simulink model "APF_Path_Planning_2023a"  (R2023a)
settings: Solver=ode4  StartTime=0.0  StopTime=tsim  FixedStep=baseRate  RelTol=1e-6  AbsTol=1e-6
values from neighbouring files (symbols this model uses):
  A = [0 0 0 1 0 0 ... (first row only)    [CTL.m]
  a = 25.028    [CTL.m]
  a1 = gain_matrix(1,1)    [CTL.m]
  alpha_m = 0.1    [CTL.m]
  alphap = 1    [CTL.m]
  alphat = 1.1    [CTL.m]
  Am = [0 0 1 0; 0 0 0 1; -wn^2 0 -2*zeta*wn 0; 0 -wn^2 0 -2*zeta*wn]    [CTL.m]
  b = gain_matrix(1,2)    [CTL.m]
  Bm = [0 0; 0 0; -wn^2 0; 0 -wn^2]    [CTL.m]
  c = gain_matrix(2,1)    [CTL.m]
  Cm = [alpha_m 0 0 0; 0 alpha_m 0 0; 0 0 1 0; 0 0 0 1]    [CTL.m]
  d = gain_matrix(2,2)    [CTL.m]
  Dm = zeros(4,2)    [CTL.m]
  epsilon = F_max/2    (= 0.11)    [CTL.m]
  F_max = 0.22    [CTL.m]
  Hz = 0.01    [CTL.m]
  J = IRED    [CTL.m]
  k = lqr(A,B1,Q,R)    [CTL.m]
  k1 = 5    [CTL.m]
  k1t = 2    [CTL.m]
  k2 = 28    [CTL.m]
  k2t = 16    [CTL.m]
  k_1_0 = 3.5    [CTL.m]
  k_1_t_0 = 1    [CTL.m]
  k_2_0 = 28    [CTL.m]
  k_2_t_0 = 1    [CTL.m]
  Kd_t = 9.5    [CTL.m]
  Kd_x = 28    [CTL.m]
  Kd_y = Kd_x    (= 28)    [CTL.m]
  Kp_t = 1    [CTL.m]
  Kp_x = 3.5    [CTL.m]
  Kp_y = Kp_x    (= 3.5)    [CTL.m]
  lambda1 = 0.4    [CTL.m]
  lambda12 = 0.4    [CTL.m]
  lambda12_t = 0.05    [CTL.m]
  lambda1_t = 0.05    [CTL.m]
  lambda2 = 0.4    [CTL.m]
  lambda2_t = 0.05    [CTL.m]
  m = mRED    [CTL.m]
  p = 0.4    [CTL.m]
  p_t = 0.05    [CTL.m]
  Q = [w 0 0 0 0 0 ... (first row only)    [CTL.m]
  R = [r 0 0 ... (first row only)    [CTL.m]
  Red_Rate = 0.025    [CTL.m]
  T_max = 0.0235    [CTL.m]
  Time_Look = 25    [CTL.m]
  xm_0 = [RED_ini(1,1:2),0,0]    [CTL.m]
undefined symbols (not defined in the file or in its folder): a2, a3, adadelta_epsilon, adadelta_gamma, adagrad_epsilon, adagrad_eta, adam_beta_1, adam_beta_2, adam_epsilon, adam_eta, adamax_beta_1, adamax_beta_2, adamax_eta, alpha, Att_Mode, b0, b1, b2, b3, baseRate, beta, Binv, BLACK_end, BLACK_ini, BLUE_end, BLUE_ini, DiscIntNeverNeededParam, drop_states_ARM, drop_states_BLACK, drop_states_BLUE, drop_states_RED, dt, end_time_black, end_time_blue, F_Black_X_nominal, F_Black_Y_nominal, F_Blue_X_nominal, F_Blue_Y_nominal, F_red_X_nominal, F_red_Y_nominal, F_thrusters_BLACK, F_thrusters_BLUE, F_thrusters_RED, Gamma1_el, Gamma1_sh, Gamma1_wr, Gamma2_el, Gamma2_sh, Gamma2_wr, Gamma3_el, Gamma3_sh, Gamma3_wr, Gamma4_el, Gamma4_sh, Gamma4_wr, Gamma5_el, Gamma5_sh, Gamma5_wr, Gamma6_el, Gamma6_sh ... (+98)
libraries: nvidiaSharedBlocks x10, MainLibrary x4, dspsigops x4, simulink x2, etargetslib x1
(part 12 of 13)

== matlab function APF_Path_Planning_2023a/Phase #3: Experiment/Change RED Behavior/Sub-Phase #4/BLACK/UKF1/MATLAB Function ==
  data: Measurments input; States output; Force input; States_k1 input; P_K1 input; P_K output; lamda parameter; J parameter; m parameter; dt parameter; Q parameter; alpha parameter; beta parameter; H parameter; R parameter; thresh parameter
function [States,P_K] = UKF(Measurments,Force,States_k1,P_K1, lamda, J, m, dt, Q, alpha, beta, H, R, thresh)
%% Block diagram got messy so i put it all in one block
if isempty(Force)
    Force = [0;0;0];
end

X_Cal= fcn1(States_k1,P_K1,lamda);

X_Cal_k1 = fcn2(Force,X_Cal,J,m,dt);

[w_m,w_c,X_tilda_k,P_K1] = fcn3(X_Cal_k1,lamda, Q, alpha, beta);

[Z_Bar,Z_Cal] = fcn4(X_Cal_k1, w_m,H);

[P_xz_k,P_z_k] = fcn5(Z_Bar,Z_Cal,w_c,X_tilda_k,X_Cal,R);

K_k = fcn6(P_xz_k,P_z_k);

Z_k = fcn7(Measurments);

Reject = fcn8(Z_k,Z_Bar,P_z_k,thresh);

States = fcn9(Z_k,Reject,X_tilda_k,Z_Bar,K_k);

P_K = fcn10(P_K1,P_z_k,K_k,Reject);
end

function X_Cal = fcn1(x_tilda_k,P_k,lamda)
%% Calculate size of sigma var
sz = 6;
N = 2*sz + 1;
X_Cal = zeros(sz,N);

%% Calculate initial sigma point
X_Cal(:,1) = x_tilda_k;

%% Calculate sigma distance
sigma = (6 + lamda)*P_k;
sigma = Cholesky_Decomposition(sigma);

%% Calculate Sigma Points
% Positive points
for i = 2:1:((N-1)/2) + 1
    fill = zeros(size(x_tilda_k));
    fill(i-1,1) = sigma(i-1,i-1);
    X_Cal(:,i) = x_tilda_k + fill;
end
% Negative Points
j = 1;
for i = N + 1 - ((N-1)/2):1:N
    fill = zeros(size(x_tilda_k));
    fill(j,1) = sigma(j,j);
    X_Cal(:,i) = x_tilda_k - fill;
    j = j + 1;
end
end

function L = Cholesky_Decomposition(mat)
%% Getting size of matrix
[row,col] = size(mat);
%% Make sure matrix can be decomposed
if row ~= col
    disp('Error due to matrix size')
    disp('Make sure square matrix is input into Cholesky Decoposition')
end

if ~isequal(size(mat), size(mat'))
    error('Input matrix must be symmetric');
end

if any(eig(mat) <= 0)
    error('Input matrix must be positive definite');
end

%% Pre allocating Space
L = zeros(row,col);

% Perform Cholesky decomposition
    for i = 1:col
        % Compute the diagonal element
        L(i, i) = sqrt(mat(i, i) - sum(L(i, 1:i-1).^2));
        
        % Compute the elements below the diagonal
        for j = i+1:col
            L(j, i) = (mat(j, i) - sum(L(j, 1:i-1).*L(i, 1:i-1))) / L(i, i);
        end
    end
end

function X_Cal_k1  = fcn2( F, X_Cal_k, J, m, dt)
%% Pre-Define
X_Cal_k1 = zeros(size(X_Cal_k));
%% System Dynamics
A = [eye(3), eye(3)*dt;
    zeros(3), eye(3)];

B = [eye(2)*(dt^2)/(2*m), zeros(2,1);
     0,0, (dt^2)/(2*J);
     eye(2)*(dt)/(m), zeros(2,1);
     0,0, (dt)/(J)];

%% State propigation
f = size(X_Cal_k,2);
for i = 1:1:f
    X_Cal_k1(:,i) = A*X_Cal_k(:,i) + B*F; 
end
end

function [w_m,w_c,X_tilda_k,P_K] = fcn3(X_Cal_k1,lamda, Q, alpha, beta)
%% Sigma weights
sz = size(X_Cal_k1,2);
N = 6;

%% For non modifyed variation
% w_0 = kappa/(N + kappa);
% w_i = 1/(2*(N + kappa));
% w = w_i*ones(1,N);
% w(1,1) = w_0;

%% Additional step - Sigma Points Weights
w_m_0 = lamda/(N + lamda);
w_c_0 = (lamda/(N + lamda)) + beta + (1 - alpha^2);
w_i = 1/(2*(N + lamda));

w = w_i*ones(1,sz-1);
w_m = [w_m_0, w];
w_c = [w_c_0, w];

w_m = diag(w_m);
w_c = diag(w_c);

%% State Prediction
X_tilda_k = X_Cal_k1*w_m;
X_tilda_k = sum(X_tilda_k,2);


%% Covariance Prediction
P_K = (X_Cal_k1 - X_tilda_k)*w_c*(X_Cal_k1 - X_tilda_k)' + Q;

end

function [Z_Bar,Z_Cal] = fcn4(x_Cal_k1, w_m,H)
%% calc Z_Cal
N = size(x_Cal_k1,2);
Z_Cal = zeros(3,N);
for i = 1:1:N
    Z_Cal(:,i) = H*x_Cal_k1(:,i);
end

%% Calc Z_Bar
Z_Bar = Z_Cal*w_m;
Z_Bar = sum(Z_Bar,2);
end

function [P_xz_k,P_z_k] = fcn5(Z_Bar,Z_Cal,w_c,x_tilda_k1,X_Cal,R)
%% calc P_z
P_z_k = (Z_Cal - Z_Bar)*w_c*(Z_Cal - Z_Bar)' + R;

%% calc P_xz
P_xz_k = (X_Cal - x_tilda_k1)*w_c*(Z_Cal - Z_Bar)';
end

function K_k = fcn6(P_xz_k,P_z_k)
K_k = (P_xz_k)*P_z_k';
end

function Z_k = fcn7(z_k)
    %% Assuming that all states are given or no states are given
    if anynan(z_k)
        Z_k = 1000*ones(3,1);
    else
    Z_k = z_k;
    end
end

function  Reject = fcn8(Z_k,Z_Bar,P_z_k,thresh)
%% Calc Mahalanobis Distance
D_square = (transpose(Z_k - Z_Bar))*P_z_k*(Z_k - Z_Bar);
% mahalanobis_d = sqrt(D_square);

%% Determine if data should be rejected
if D_square < thresh
    Reject = 0;
else
    Reject = 1;
end
end

function [x] = fcn9(z,Reject,X_tilda_k,z_bar,K_k)
%% State estimate
    if Reject == 0
        x = X_tilda_k + K_k*(z - z_bar);
    else
        x = X_tilda_k;
    end
end

function P_K = fcn10(P_k1,P_z_k,K_k,Reject)
if Reject == 0
    P_K = P_k1 - (K_k*P_z_k)*K_k';
else
    P_K = P_k1;
end
end

== matlab function APF_Path_Planning_2023a/Phase #3: Experiment/Change BLUE Behavior/Sub-Phase #3 /Hough Control/MATLAB Function2 ==
  data: Oy output; z input; Ox output
function [Oy, Ox]   = C3( z )
%C3 gives the rotation matrix about the z-axis for an angle 'z'
%   z - the angle about the z-axis which you rotate
%   A - the rotation matrix

Ox = [cos(z) sin(z); -sin(z) cos(z)]*[1;0];
Oy = [cos(z) sin(z); -sin(z) cos(z)]*[0;1];
end

== matlab function APF_Path_Planning_2023a/Phase #3: Experiment/Change BLUE Behavior/Sub-Phase #3 /Hough Control/MATLAB Function3 ==
  data: z input; Ox output
function Ox    = C3( z )
%C3 gives the rotation matrix about the z-axis for an angle 'z'
%   z - the angle about the z-axis which you rotate
%   A - the rotation matrix

Ox = [cos(z) sin(z); -sin(z) cos(z)]*[1;0];
end

== matlab function APF_Path_Planning_2023a/Phase #3: Experiment/Change BLUE Behavior/Sub-Phase #3 /Hough Control/MATLAB Function4 ==
  data: Oy input; e_out output; e_in input
function e_out = fcn(Oy, e_in)

a = sign(Oy'*e_in);
e_out = -a*norm(e_in);

== matlab function APF_Path_Planning_2023a/Phase #3: Experiment/Change BLUE Behavior/Sub-Phase #3 /MATLAB Function2 ==
  data: t input; x output; xLength parameter
function x = fcn(t, xLength)

x = -0.85*cos((0.03490659)*t) + xLength/2;

end

== matlab function APF_Path_Planning_2023a/Phase #3: Experiment/Change BLUE Behavior/Sub-Phase #3 /MATLAB Function3 ==
  data: t input; y output; yLength parameter
function y = fcn(t, yLength)

y = -0.85*sin((0.03490659)*t) + yLength/2;

end

== matlab function APF_Path_Planning_2023a/Phase #5: Hold Home/Change BLUE Behavior/Hough Control/MATLAB Function4 ==
  data: Oy input; e_out output; e_in input
function e_out = fcn(Oy, e_in)

a = sign(Oy'*e_in);
e_out = -a*norm(e_in);

== matlab function APF_Path_Planning_2023a/Phase #3: Experiment/Change RED Behavior/Sub-Phase #4/BLACK/Parker's Transform ==
  data: rel_state_black input; state_red input; abs_state_black output
function abs_state_black = fcn(rel_state_black,state_red)
%calcualtes ECI pos/att of black

% messing with rel state black
rel_state_black(1) = rel_state_black(1)/100;
rel_state_black(2) = rel_state_black(2)/100;
rel_state_black(3) = rel_state_black(3)*(pi/180)+pi/2; 

angle = -state_red(3);

C = [cos(angle),sin(angle);
     -sin(angle),cos(angle)];

abs_distance_black = C*[rel_state_black(1);rel_state_black(2)];

abs_pos_black = [state_red(1);state_red(2)] + abs_distance_black;

abs_angle_black = rel_state_black(3) - state_red(3);

abs_state_black =  [abs_pos_black;
                    abs_angle_black];

== matlab function APF_Path_Planning_2023a/Phase #3: Experiment/Change RED Behavior/Sub-Phase #4/BLACK/Kalman Filter1/MATLAB Function ==
  data: z_k input; Z_k output
function Z_k = fcn(z_k)
    %% Assuming that all states are given or no states are given
    if anynan(z_k)
        Z_k = zeros(3,1);
    else
    Z_k = z_k;
    end
end

== matlab function APF_Path_Planning_2023a/Phase #3: Experiment/Change RED Behavior/Sub-Phase #4/BLACK/Kalman Filter1/MATLAB Function1 ==
  data: P_k input; P_k1 output; A parameter; Q_T parameter
function P_k1 = fcn(P_k,A, Q_T)
if isempty(P_k) 
    P_k1 = Peye(6);
else
    P_k1 = A*P_k*(transpose(A)) + Q_T;
end
end

== matlab function APF_Path_Planning_2023a/Phase #3: Experiment/Change RED Behavior/Sub-Phase #4/BLACK/Kalman Filter1/MATLAB Function2 ==
  data: P_k1 input; K_k output; H parameter; R parameter
function K_k = fcn(P_k1,H, R)

K_k = P_k1*(transpose(H))/(H*P_k1*(transpose(H)) + R);
end

== matlab function APF_Path_Planning_2023a/Phase #3: Experiment/Change RED Behavior/Sub-Phase #4/BLACK/Kalman Filter1/MATLAB Function3 ==
  data: P_k1 input; P_K output; K_k input; H parameter
function P_K = fcn(P_k1,K_k,H)
P_K = zeros(6,6);
P_K = P_k1 - (K_k*H*P_k1); 
end

== matlab function APF_Path_Planning_2023a/Phase #3: Experiment/Change RED Behavior/Sub-Phase #4/BLACK/Kalman Filter1/MATLAB Function4 ==
  data: Z_k input; x output; X_tilda_k input; K_k input; H parameter
function x = fcn(Z_k,X_tilda_k,K_k,H)

x = X_tilda_k + K_k*(Z_k - H*X_tilda_k);
end

== matlab function APF_Path_Planning_2023a/Phase #3: Experiment/Change RED Behavior/Sub-Phase #4/BLACK/Kalman Filter1/MATLAB Function5 ==
  data: X_tilda_k1 input; x_tilda_k output; A parameter
function x_tilda_k = fcn(X_tilda_k1,A)

x_tilda_k = A*X_tilda_k1;
end

== matlab function APF_Path_Planning_2023a/Phase #3: Experiment/Change RED Behavior/Sub-Phase #4/CTL/Target Tracker/LQR1/MATLAB Function ==
  data: k input; u output; q1_x input; q2_x input; q1_y input; q2_y input; q1_t input; q2_t input
function u = fcn(k,q1_x,q2_x,q1_y,q2_y,q1_t,q2_t)

x = [q1_x;
    q1_y;
    q1_t;
    q2_x;
    q2_y;
    q2_t];

u = k*x;
% u = [0; 0; 0];

== matlab function APF_Path_Planning_2023a/Phase #3: Experiment/Change RED Behavior/Sub-Phase #4/CTL/If Action Subsystem/CSMC3/MATLAB Function ==
  data: phi input; u output; alphap parameter
function u = fcn(phi, alphap)



u = sign(phi)*(abs(phi)^(alphap/(2 - alphap)));

== matlab function APF_Path_Planning_2023a/Phase #5: Hold Home/Change RED Behavior/Hough Control/MATLAB Function2 ==
  data: Oy output; z input; Ox output
function [Oy, Ox]   = C3( z )
%C3 gives the rotation matrix about the z-axis for an angle 'z'
%   z - the angle about the z-axis which you rotate
%   A - the rotation matrix

Ox = [cos(z) sin(z); -sin(z) cos(z)]*[1;0];
Oy = [cos(z) sin(z); -sin(z) cos(z)]*[0;1];
end

== matlab function APF_Path_Planning_2023a/Phase #3: Experiment/Change RED Behavior/Sub-Phase #4/GDC/Target Finder/Constant Angular Rate/Wrap1/MATLAB Function ==
  data: u input; wrappedAngle output
function wrappedAngle = wrapAngle(u)

wrappedAngle = atan2(sin(u),cos(u));

end

== matlab function APF_Path_Planning_2023a/Phase #3: Experiment/Change RED Behavior/Sub-Phase #4/CTL/If Action Subsystem/CSMC3/MATLAB Function1 ==
  data: q2 input; u output; k1 parameter; alphap parameter
function u = fcn(q2,k1, alphap)

u = sign(k1*q2)*(abs(k1*q2)^alphap);

== matlab function APF_Path_Planning_2023a/Phase #3: Experiment/Change RED Behavior/Sub-Phase #4/CTL/If Action Subsystem/CSMC3/MATLAB Function2 ==
  data: q1 input; phi output; k1 parameter; alphap parameter; q2 input
function phi = fcn(q1,k1, alphap, q2)



phi = k1*q1 + (1/(2 - alphap))*sign(k1*q2)*(abs(k1*q2))^(2 - alphap);

== matlab function APF_Path_Planning_2023a/Phase #3: Experiment/Change RED Behavior/Sub-Phase #4/CTL/If Action Subsystem/CSMC3/MATLAB Function3 ==
  data: phi input; u output; alphap parameter
function u = fcn(phi, alphap)



u = sign(phi)*(abs(phi)^(alphap/(2 - alphap)));

== matlab function APF_Path_Planning_2023a/Phase #3: Experiment/Change RED Behavior/Sub-Phase #4/CTL/If Action Subsystem/CSMC3/MATLAB Function4 ==
  data: q2 input; u output; k1 parameter; alphap parameter
function u = fcn(q2,k1, alphap)

u = sign(k1*q2)*(abs(k1*q2)^alphap);

== matlab function APF_Path_Planning_2023a/Phase #3: Experiment/Change RED Behavior/Sub-Phase #4/CTL/If Action Subsystem/CSMC3/MATLAB Function5 ==
  data: q1 input; phi output; k1 parameter; alphap parameter; q2 input
function phi = fcn(q1,k1, alphap, q2)



phi = k1*q1 + (1/(2 - alphap))*sign(k1*q2)*(abs(k1*q2))^(2 - alphap);

== matlab function APF_Path_Planning_2023a/Phase #3: Experiment/Change RED Behavior/Sub-Phase #4/CTL/If Action Subsystem/CSMC3/MATLAB Function6 ==
  data: phi input; u output; alpha parameter
function u = fcn(phi, alpha)



u = sign(phi)*(abs(phi)^(alpha/(2 - alpha)));

== matlab function APF_Path_Planning_2023a/Phase #3: Experiment/Change RED Behavior/Sub-Phase #4/CTL/If Action Subsystem/CSMC3/MATLAB Function7 ==
  data: q2 input; u output; k1 parameter; alpha parameter
function u = fcn(q2,k1, alpha)

u = sign(k1*q2)*(abs(k1*q2)^alpha);

== matlab function APF_Path_Planning_2023a/Phase #3: Experiment/Change RED Behavior/Sub-Phase #4/CTL/If Action Subsystem/CSMC3/MATLAB Function8 ==
  data: q1 input; phi output; k1 parameter; alpha parameter; q2 input
function phi = fcn(q1,k1, alpha, q2)



phi = k1*q1 + (1/(2 - alpha))*sign(k1*q2)*(abs(k1*q2))^(2 - alpha);

== matlab function APF_Path_Planning_2023a/Phase #5: Hold Home/Change RED Behavior/Hough Control/MATLAB Function3 ==
  data: z input; Ox output
function Ox    = C3( z )
%C3 gives the rotation matrix about the z-axis for an angle 'z'
%   z - the angle about the z-axis which you rotate
%   A - the rotation matrix

Ox = [cos(z) sin(z); -sin(z) cos(z)]*[1;0];
end

== matlab function APF_Path_Planning_2023a/Phase #3: Experiment/Change RED Behavior/Sub-Phase #4/CTL/If Action Subsystem/DAC Controller2/Fx Gain Derivatives ==
  data: e_xdot input; k2_dot output; e_x input; k1_dot output; lambda1 parameter; lambda2 parameter; lambda12 parameter; p parameter
function [k2_dot, k1_dot]= fcn(e_xdot, e_x, lambda1, lambda2, lambda12, p)

k1_dot = -lambda1*p*e_x^2-(lambda1+p*lambda12)*e_x*e_xdot-lambda12*e_xdot^2;
k2_dot = -lambda12*p*e_x^2-(lambda12+p*lambda2)*e_x*e_xdot-lambda2*e_xdot^2;

== matlab function APF_Path_Planning_2023a/Phase #3: Experiment/Change RED Behavior/Sub-Phase #4/CTL/If Action Subsystem/DAC Controller2/Fy Gain Derivatives ==
  data: k2_dot output; e_ydot input; e_y input; k1_dot output; lambda1 parameter; lambda2 parameter; lambda12 parameter; p parameter
function [k2_dot, k1_dot]= fcn(e_ydot, e_y, lambda1, lambda2, lambda12, p)

k1_dot = -lambda1*p*e_y^2-(lambda1+p*lambda12)*e_y*e_ydot-lambda12*e_ydot^2;
k2_dot = -lambda12*p*e_y^2-(lambda12+p*lambda2)*e_y*e_ydot-lambda2*e_ydot^2;

== matlab function APF_Path_Planning_2023a/Phase #3: Experiment/Change RED Behavior/Sub-Phase #4/CTL/If Action Subsystem/DAC Controller2/Torque Gain Derivatives ==
  data: e_t input; e_tdot input; k1_dot output size=1; k2_dot output size=1; lambda1_t parameter; lambda2_t parameter; lambda12_t parameter; p_t parameter
function [k1_dot, k2_dot]= fcn(e_t, e_tdot, lambda1_t, lambda2_t, lambda12_t, p_t)
k1_dot = -lambda1_t*p_t*e_t^2-(lambda1_t+p_t*lambda12_t)*e_t*e_tdot-lambda12_t*e_tdot^2;
k2_dot = -lambda12_t*p_t*e_t^2-(lambda12_t+p_t*lambda2_t)*e_t*e_tdot-lambda2_t*e_tdot^2;

== matlab function APF_Path_Planning_2023a/Phase #3: Experiment/Change RED Behavior/Sub-Phase #4/CTL/If Action Subsystem/Homo/MATLAB Function ==
  data: q1 input; u output; k1 parameter; alphap parameter
function u = fcn(q1,k1, alphap)

u = k1*sign(q1)*(abs(q1)^(alphap/(2 - alphap)));

== matlab function APF_Path_Planning_2023a/Phase #3: Experiment/Change RED Behavior/Sub-Phase #4/CTL/If Action Subsystem/Homo/MATLAB Function1 ==
  data: q2 input; u output; k2 parameter; alphap parameter
function u = fcn(q2,k2, alphap)

u = k2*sign(q2)*(abs(q2)^alphap);

== matlab function APF_Path_Planning_2023a/Phase #3: Experiment/Change RED Behavior/Sub-Phase #4/CTL/If Action Subsystem/DAC Controller1/Fy Gain Derivatives ==
  data: k2_dot output; e_ydot input; e_y input; k1_dot output; lambda1 parameter; lambda2 parameter; lambda12 parameter; p parameter
function [k2_dot, k1_dot]= fcn(e_ydot, e_y, lambda1, lambda2, lambda12, p)

k1_dot = -lambda1*p*e_y^2-(lambda1+p*lambda12)*e_y*e_ydot-lambda12*e_ydot^2;
k2_dot = -lambda12*p*e_y^2-(lambda12+p*lambda2)*e_y*e_ydot-lambda2*e_ydot^2;

== matlab function APF_Path_Planning_2023a/Phase #5: Hold Home/Change RED Behavior/Hough Control/MATLAB Function4 ==
  data: Oy input; e_out output; e_in input
function e_out = fcn(Oy, e_in)

a = sign(Oy'*e_in);
e_out = -a*norm(e_in);

== matlab function APF_Path_Planning_2023a/Phase #3: Experiment/Change RED Behavior/Sub-Phase #4/CTL/If Action Subsystem/DAC Controller1/Torque Gain Derivatives ==
  data: e_t input; e_tdot input; k1_dot output size=1; k2_dot output size=1; lambda1_t parameter; lambda2_t parameter; lambda12_t parameter; p_t parameter
function [k1_dot, k2_dot]= fcn(e_t, e_tdot, lambda1_t, lambda2_t, lambda12_t, p_t)
k1_dot = -lambda1_t*p_t*e_t^2-(lambda1_t+p_t*lambda12_t)*e_t*e_tdot-lambda12_t*e_tdot^2;
k2_dot = -lambda12_t*p_t*e_t^2-(lambda12_t+p_t*lambda2_t)*e_t*e_tdot-lambda2_t*e_tdot^2;

== matlab function APF_Path_Planning_2023a/Phase #3: Experiment/Change RED Behavior/Sub-Phase #4/CTL/If Action Subsystem/Homo/MATLAB Function4 ==
  data: q1 input; u output; k1t parameter; alphat parameter
function u = fcn(q1,k1t, alphat)

u = k1t*sign(q1)*(abs(q1)^(alphat/(2 - alphat)));

== matlab function APF_Path_Planning_2023a/Phase #3: Experiment/Change RED Behavior/Sub-Phase #4/CTL/If Action Subsystem/Homo/MATLAB Function5 ==
  data: q2 input; u output; k2t parameter; alphat parameter
function u = fcn(q2,k2t, alphat)

u = k2t*sign(q2)*(abs(q2)^alphat);

== matlab function APF_Path_Planning_2023a/Phase #3: Experiment/Change RED Behavior/Sub-Phase #4/CTL/If Action Subsystem/LQR/MATLAB Function ==
  data: k input; u output; q1_x input; q2_x input; q1_y input; q2_y input; q1_t input; q2_t input
function u = fcn(k,q1_x,q2_x,q1_y,q2_y,q1_t,q2_t)

x = [q1_x;
    q1_y;
    q1_t;
    q2_x;
    q2_y;
    q2_t];

u = k*x;
% u = [0; 0; 0];

== matlab function APF_Path_Planning_2023a/Phase #3: Experiment/Change RED Behavior/Sub-Phase #4/CTL/If Action Subsystem/Sat/MATLAB Function ==
  data: q2 input; q1 input; saturation output; a1 parameter; b parameter; m parameter
function saturation = fcn(q2,q1,a1, b, m)

u = a1*m*q1 + a1*m*q2/b;

saturation = u;

== matlab function APF_Path_Planning_2023a/Phase #3: Experiment/Change RED Behavior/Sub-Phase #4/CTL/If Action Subsystem/Sat/MATLAB Function1 ==
  data: q2 input; q1 input; saturation output; a1 parameter; b parameter; m parameter
function saturation = fcn(q2,q1,a1, b, m)

u = a1*m*q1 + a1*m*q2/b;

saturation = u;

== matlab function APF_Path_Planning_2023a/Phase #3: Experiment/Change RED Behavior/Sub-Phase #4/CTL/If Action Subsystem/Sat/MATLAB Function2 ==
  data: q2 input; q1 input; saturation output; c parameter; d parameter; J parameter
function saturation = fcn(q2,q1,c, d, J)

u = c*J*q1 + c*J*q2/d;

saturation = u;

== matlab function APF_Path_Planning_2023a/Simulate Plant Dynamics/RED and ARM Dynamics/RED + ARM/RED + ARM Dynamics/Coriolis Function1 ==
  data: a1 parameter; a2 parameter; a3 parameter; b0 parameter; b1 parameter; b2 parameter; mPROX parameter; mDIST parameter; mEE parameter; Phi parameter; CoriolisS output; x input
function CoriolisS = CoriolisFunc3LINK(a1,a2,a3,b0,b1,b2,mPROX,mDIST,mEE,Phi,x)
%CORIOLISFUNC3LINK
%    CORIOLISS = CORIOLISFUNC3LINK(A1,A2,A3,B0,B1,B2,mPROX,mDIST,mEE,PHI,Q0,Q1,Q2,Q3,Q0_DOT,Q1_DOT,Q2_DOT,Q3_DOT)

%    This function was generated by the Symbolic Math Toolbox version 8.0.
%    05-Nov-2017 11:48:44

q0 = x(3);
q1 = x(4);
q2 = x(5);
q3 = x(6);

q0_dot = x(9);
q1_dot = x(10);
q2_dot = x(11);
q3_dot = x(12);

t2 = a1+b1;
t3 = a1.*mPROX;
t4 = mDIST.*t2;
t5 = mEE.*t2;
t6 = t3+t4+t5;
t7 = a2.*mDIST;
t8 = a2+b2;
t9 = mEE.*t8;
t10 = t7+t9;
t11 = pi.*(1.0./2.0);
t12 = q0_dot.*t6;
t13 = q1_dot.*t6;
t14 = q0+q1+t11;
t15 = cos(t14);
t16 = t12+t13;
t17 = q0_dot.*t10;
t18 = q1_dot.*t10;
t19 = q2_dot.*t10;
t20 = q0+q1+q2+t11;
t21 = cos(t20);
t22 = t17+t18+t19;
t23 = a3.*mEE.*q0_dot;
t24 = a3.*mEE.*q1_dot;
t25 = a3.*mEE.*q2_dot;
t26 = a3.*mEE.*q3_dot;
t27 = q0+q1+q2+q3+t11;
t28 = cos(t27);
t29 = t23+t24+t25+t26;
t30 = b0.*mPROX;
t31 = b0.*mDIST;
t32 = b0.*mEE;
t33 = t30+t31+t32;
t34 = (pi/2-Phi)+q0;
t35 = sin(t14);
t36 = sin(t20);
t37 = sin(t27);
t38 = q0_dot+q1_dot+q2_dot+q3_dot;
t39 = q0+q1+q2+q3;
t40 = a1.*b0.*mPROX.*q1_dot;
t41 = a1.*b0.*mDIST.*q1_dot;
t42 = a1.*b0.*mEE.*q1_dot;
t43 = b0.*b1.*mDIST.*q1_dot;
t44 = b0.*b1.*mEE.*q1_dot;
t45 = (pi/2-Phi)-q1;
t46 = cos(t45);
t47 = a2.*b0.*mDIST.*q1_dot;
t48 = a2.*b0.*mDIST.*q2_dot;
t49 = a2.*b0.*mEE.*q1_dot;
t50 = a2.*b0.*mEE.*q2_dot;
t51 = b0.*b2.*mEE.*q1_dot;
t52 = b0.*b2.*mEE.*q2_dot;
t53 = -(pi/2-Phi)+q1+q2;
t54 = cos(t53);
t55 = a3.*b0.*mEE.*q1_dot;
t56 = a3.*b0.*mEE.*q2_dot;
t57 = a3.*b0.*mEE.*q3_dot;
t58 = -(pi/2-Phi)+q1+q2+q3;
t59 = cos(t58);
t60 = a2.*b1.*mDIST.*q2_dot;
t61 = a1.*b2.*mEE.*q2_dot;
t62 = a2.*b1.*mEE.*q2_dot;
t63 = b1.*b2.*mEE.*q2_dot;
t64 = a1.*a2.*mDIST.*q2_dot;
t65 = a1.*a2.*mEE.*q2_dot;
t66 = sin(q2);
t67 = t60+t61+t62+t63+t64+t65;
t68 = a3.*b2.*mEE.*q3_dot;
t69 = a2.*a3.*mEE.*q3_dot;
t70 = sin(q3);
t71 = t68+t69;
t72 = a3.*b1.*mEE.*q2_dot;
t73 = a3.*b1.*mEE.*q3_dot;
t74 = a1.*a3.*mEE.*q2_dot;
t75 = a1.*a3.*mEE.*q3_dot;
t76 = q2+q3;
t77 = sin(t76);
t78 = t72+t73+t74+t75;
t79 = a2.*b0.*mDIST.*q0_dot;
t80 = a2.*b0.*mEE.*q0_dot;
t81 = b0.*b2.*mEE.*q0_dot;
t82 = t47+t48+t49+t50+t51+t52+t79+t80+t81;
t83 = a3.*b0.*mEE.*q0_dot;
t84 = t55+t56+t57+t83;
t85 = a1.*b0.*mPROX.*q0_dot;
t86 = a1.*b0.*mDIST.*q0_dot;
t87 = a1.*b0.*mEE.*q0_dot;
t88 = b0.*b1.*mDIST.*q0_dot;
t89 = b0.*b1.*mEE.*q0_dot;
t90 = a2.*b1.*mDIST.*q0_dot;
t91 = a1.*b2.*mEE.*q0_dot;
t92 = a2.*b1.*mDIST.*q1_dot;
t93 = a2.*b1.*mEE.*q0_dot;
t94 = a1.*b2.*mEE.*q1_dot;
t95 = a2.*b1.*mEE.*q1_dot;
t96 = b1.*b2.*mEE.*q0_dot;
t97 = b1.*b2.*mEE.*q1_dot;
t98 = a1.*a2.*mDIST.*q0_dot;
t99 = a1.*a2.*mDIST.*q1_dot;
t100 = a1.*a2.*mEE.*q0_dot;
t101 = a1.*a2.*mEE.*q1_dot;
t102 = t60+t61+t62+t63+t64+t65+t90+t91+t92+t93+t94+t95+t96+t97+t98+t99+t100+t101;
t103 = a3.*b1.*mEE.*q0_dot;
t104 = a3.*b1.*mEE.*q1_dot;
t105 = a1.*a3.*mEE.*q0_dot;
t106 = a1.*a3.*mEE.*q1_dot;
t107 = t72+t73+t74+t75+t103+t104+t105+t106;
t108 = t79+t80+t81;
t109 = t54.*t108;
t110 = t59.*t83;
t111 = t90+t91+t92+t93+t94+t95+t96+t97+t98+t99+t100+t101;
t112 = t66.*t111;
t113 = t103+t104+t105+t106;
t114 = t77.*t113;
t115 = a2.*q0_dot;
t116 = a2.*q1_dot;
t117 = a2.*q2_dot;
t118 = b2.*q0_dot;
t119 = b2.*q1_dot;
t120 = b2.*q2_dot;
t121 = t115+t116+t117+t118+t119+t120;
t122 = a3.*mEE.*t70.*t121;
t123 = a1.*q0_dot;
t124 = a1.*q1_dot;
t125 = b1.*q0_dot;
t126 = b1.*q1_dot;
t127 = t123+t124+t125+t126;
t128 = a3.*mEE.*t77.*t127;
CoriolisS = reshape([0.0,0.0,0.0,0.0,0.0,0.0,0.0,0.0,0.0,0.0,0.0,0.0,-t15.*t16-t21.*t22-t28.*t29-q0_dot.*t33.*cos(t34),-t16.*t35-t22.*t36-t29.*t37-q0_dot.*t33.*sin(t34),-t66.*t67-t70.*t71-t77.*t78-t46.*(t40+t41+t42+t43+t44)-t59.*(t55+t56+t57)-t54.*(t47+t48+t49+t50+t51+t52),t109+t110-t66.*t67-t70.*t71-t77.*t78+t46.*(t85+t86+t87+t88+t89),t109+t110+t112+t114-t70.*t71,t110+t122+t128,-t15.*t16-t21.*t22-t28.*t29,-t16.*t35-t22.*t36-t29.*t37,-t66.*t67-t54.*t82-t70.*t71-t59.*t84-t77.*t78-t46.*(t40+t41+t42+t43+t44+t85+t86+t87+t88+t89),-t66.*t67-t70.*t71-t77.*t78,t112+t114-t70.*t71,t122+t128,-t21.*t22-t28.*t29,-t22.*t36-t29.*t37,-t54.*t82-t70.*t71-t59.*t84-t66.*t102-t77.*t107,-t70.*t71-t66.*t102-t77.*t107,-a3.*mEE.*q3_dot.*t8.*t70,a3.*mEE.*t8.*t70.*(q0_dot+q1_dot+q2_dot),a3.*mEE.*t38.*sin(t39),-a3.*mEE.*t38.*cos(t39),-a3.*b0.*mEE.*t38.*t59-a3.*mEE.*t8.*t38.*t70-a3.*mEE.*t2.*t38.*t77,-a3.*mEE.*t8.*t38.*t70-a3.*mEE.*t2.*t38.*t77,-a3.*mEE.*t8.*t38.*t70,0.0],[6,6]);
end

== matlab function APF_Path_Planning_2023a/Phase #3: Experiment/Change RED Behavior/Sub-Phase #4/CTL/If Action Subsystem/Sat/MATLAB Function3 ==
  data: q2 input; u input; saturation output; F_max parameter; e parameter; b parameter; m parameter
function saturation = fcn(q2,u,F_max, e, b, m)

if u >= e
    u = e;
elseif u <= -1*e
    u = -1*e;
else
    u = u;
end

u = b*q2*m + u;

if u >= F_max
    u = F_max;
elseif u <= -1*F_max
    u = -1*F_max;
else
    u = u;
end

saturation = u;

== matlab function APF_Path_Planning_2023a/Phase #3: Experiment/Change RED Behavior/Sub-Phase #4/CTL/If Action Subsystem/Sat/MATLAB Function4 ==
  data: q2 input; u input; saturation output; F_max parameter; b parameter; m parameter; e parameter
function saturation = fcn(q2,u,F_max, b, m, e)

if u >= e
    u = e;
elseif u <= -1*e
    u = -1*e;
else
    u = u;
end

u = b*q2*m + u;

if u >= F_max
    u = F_max;
elseif u <= -1*F_max
    u = -1*F_max;
else
    u = u;
end

saturation = u;

== matlab function APF_Path_Planning_2023a/Phase #3: Experiment/Change RED Behavior/Sub-Phase #4/CTL/If Action Subsystem/Sat/MATLAB Function5 ==
  data: q2 input; u input; saturation output; e parameter; T_max parameter; d parameter; J parameter
function saturation = fcn(q2,u,e, T_max, d, J)

if u >= e
    u = e;
elseif u <= -1*e
    u = -1*e;
else
    u = u;
end

u = d*q2*J + u;

if u >= T_max
    u = T_max;
elseif u <= -1*T_max
    u = -1*T_max;
else
    u = u;
end

saturation = u;

== matlab function APF_Path_Planning_2023a/Phase #3: Experiment/Change RED Behavior/Sub-Phase #4/CTL/Subsystem1/SAT_Angle1/MATLAB Function2 ==
  data: q2 input; q1 input; saturation output; c parameter; d parameter; J parameter
function saturation = fcn(q2,q1,c, d, J)

u = c*J*q1 + c*J*q2/d;

saturation = u;

== matlab function APF_Path_Planning_2023a/Phase #3: Experiment/Change RED Behavior/Sub-Phase #4/CTL/Subsystem1/SAT_Angle1/MATLAB Function5 ==
  data: q2 input; u input; saturation output; e parameter; T_max parameter; d parameter; J parameter
function saturation = fcn(q2,u,e, T_max, d, J)

if u >= e
    u = e;
elseif u <= -1*e
    u = -1*e;
else
    u = u;
end

u = d*q2*J + u;

if u >= T_max
    u = T_max;
elseif u <= -1*T_max
    u = -1*T_max;
else
    u = u;
end

saturation = u;

== matlab function APF_Path_Planning_2023a/Phase #3: Experiment/Change RED Behavior/Sub-Phase #4/CTL/Subsystem1/Subsystem/SAC Ctl/SAC Fns ==
  data: um input; u output; xm input; ey input; Ke_l input; Kx_l input; Ku_l input; Ke output; Kx output; Ku output; Kedot_l output; Kxdot_l output; Kudot_l output
function [u, Ke, Kx, Ku, Kedot_l, Kxdot_l, Kudot_l] = sac(um, xm, ey, Ke_l, Kx_l, Ku_l)

%%% Gains
gamma_l = [451300 0 0; 0 0 0; 0 0 0] ;
gamma_p = 3.5*[122500 0 0; 0 534500 0; 0 0 258000] ;
sigma_sac = 0.93 ;

%%% Ke
Kpe = ey*ey'*gamma_p(1,1) ;
Kedot_l = ey*ey'*gamma_l(1,1) - sigma_sac*Ke_l ;
Ke = Kpe + Ke_l ;

%%% Kx
Kpx = ey*xm'*gamma_p(2,2) ;
Kxdot_l = ey*xm'*gamma_l(2,2) ;
Kx = Kpx + Kx_l ;

%%% Ku
Kpu = ey*um'*gamma_p(3,3) ;
Kudot_l = ey*um'*gamma_l(3,3) ;
Ku = Kpu + Ku_l ;

%%% input
u = Ke*ey + Kx*xm + Ku*um ;

== matlab function APF_Path_Planning_2023a/Phase #3: Experiment/Change RED Behavior/Sub-Phase #4/CTL/Subsystem1/SAT_Angle1/Torque Gain Derivatives ==
  data: e_t input; e_tdot input; k1_dot output size=1; k2_dot output size=1; lambda1_t parameter; lambda2_t parameter; lambda12_t parameter; p_t parameter
function [k1_dot, k2_dot]= fcn(e_t, e_tdot, lambda1_t, lambda2_t, lambda12_t, p_t)
k1_dot = -lambda1_t*p_t*e_t^2-(lambda1_t+p_t*lambda12_t)*e_t*e_tdot-lambda12_t*e_tdot^2;
k2_dot = -lambda12_t*p_t*e_t^2-(lambda12_t+p_t*lambda2_t)*e_t*e_tdot-lambda2_t*e_tdot^2;

== matlab function APF_Path_Planning_2023a/Thruster Control Code/Change RED Behavior/Calculate Thruster ON//OFF/MATLAB Function11 ==
  data: H output; thruster_dist2CG_RED parameter; F_red_X_nominal parameter; thrust_decay_factor input; F_red_Y_nominal parameter
function H   = MakeHWithDecay(thruster_dist2CG_RED,F_red_X_nominal, thrust_decay_factor, F_red_Y_nominal)


adjusted_thruster_dist2CG_RED = [thruster_dist2CG_RED(1);
                                 thruster_dist2CG_RED(2);
                                 thruster_dist2CG_RED(3);
                                 thruster_dist2CG_RED(4);
                                 thruster_dist2CG_RED(5);
                                 thruster_dist2CG_RED(6);
                                 thruster_dist2CG_RED(7);
                                 thruster_dist2CG_RED(8)];
                                 


Vec1 = [ -1
         -1
          0 
          0
          1
          1
          0
          0 ];
      
Vec2 = [  0
          0
          1
          1
          0
          0
         -1
         -1 ];
     
Vec3 = adjusted_thruster_dist2CG_RED./1000;

Mat1 = [Vec1, Vec2, Vec3]';

F_thrusters_RED = [F_red_X_nominal*thrust_decay_factor; F_red_X_nominal*thrust_decay_factor; F_red_Y_nominal*thrust_decay_factor; F_red_Y_nominal*thrust_decay_factor; F_red_X_nominal*thrust_decay_factor; F_red_X_nominal*thrust_decay_factor; F_red_Y_nominal*thrust_decay_factor; F_red_Y_nominal*thrust_decay_factor];

Mat2 = diag((F_thrusters_RED./2));

H    = Mat1*Mat2;

end

== matlab function APF_Path_Planning_2023a/Simulate Plant Dynamics/RED and ARM Dynamics/RED + ARM/RED + ARM Dynamics/Inertia Function 1 ==
  data: mRED parameter; IRED parameter; Phi parameter; b0 parameter; a1 parameter; b1 parameter; a2 parameter; b2 parameter; a3 parameter; b3 parameter; mPROX parameter; mDIST parameter; mEE parameter; IPROX parameter; IDIST parameter; InertiaS output; x input; IEE parameter
function InertiaS = InertiaFunc3LINK(mRED, IRED, Phi, b0, a1, b1, a2, b2, a3, b3, mPROX, mDIST, mEE, IPROX, IDIST, x, IEE)

    q0 = x(3);
    q1 = x(4);
    q2 = x(5);
    q3 = x(6);
    
    t2 = a1+b1;
    t3 = a1.*mPROX;
    t4 = mDIST.*t2;
    t5 = mEE.*t2;
    t6 = q0+q1;
    t7 = cos(t6);
    t8 = t3+t4+t5;
    t9 = a2.*mDIST;
    t10 = a2+b2;
    t11 = mEE.*t10;
    t12 = q0+q1+q2;
    t13 = cos(t12);
    t14 = t9+t11;
    t15 = q0+q1+q2+q3;
    t16 = cos(t15);
    t17 = mRED+mPROX+mDIST+mEE;
    t18 = b0.*mPROX;
    t19 = b0.*mDIST;
    t20 = b0.*mEE;
    t21 = t18+t19+t20;
    t22 = (pi/2-Phi)+q0;
    t23 = sin(t6);
    t24 = sin(t12);
    t25 = sin(t15);
    t26 = a2.*mEE;
    t27 = b2.*mEE;
    t28 = t9+t26+t27;
    t29 = sin(t22);
    t86 = t7.*t8;
    t87 = t13.*t14;
    t88 = a3.*mEE.*t16;
    t30 = -t86-t87-t88-t21.*t29;
    t31 = cos(t22);
    t32 = t21.*t31;
    t89 = t8.*t23;
    t90 = t14.*t24;
    t91 = a3.*mEE.*t25;
    t33 = t32-t89-t90-t91;
    t34 = a1.^2;
    t35 = a2.^2;
    t36 = b0.^2;
    t37 = b1.^2;
    t38 = a1.*a2.*mDIST.*2.0;
    t39 = a1.*a2.*mEE.*2.0;
    t40 = a2.*b1.*mDIST.*2.0;
    t41 = a1.*b2.*mEE.*2.0;
    t42 = a2.*b1.*mEE.*2.0;
    t43 = b1.*b2.*mEE.*2.0;
    t44 = t38+t39+t40+t41+t42+t43;
    t45 = cos(q2);
    t46 = t44.*t45;
    t47 = a2.*a3.*mEE.*2.0;
    t48 = a3.*b2.*mEE.*2.0;
    t49 = t47+t48;
    t50 = cos(q3);
    t51 = t49.*t50;
    t52 = a1.*a3.*mEE.*2.0;
    t53 = a3.*b1.*mEE.*2.0;
    t54 = t52+t53;
    t55 = q2+q3;
    t56 = cos(t55);
    t57 = t54.*t56;
    t58 = (pi/2-Phi)-q1;
    t59 = sin(t58);
    t60 = -(pi/2-Phi)+q1+q2;
    t61 = sin(t60);
    t62 = -(pi/2-Phi)+q1+q2+q3;
    t63 = sin(t62);
    t64 = mPROX.*t34;
    t65 = mDIST.*t34;
    t66 = mEE.*t34;
    t67 = mDIST.*t35;
    t68 = mEE.*t35;
    t69 = a3.^2;
    t70 = mEE.*t69;
    t71 = mDIST.*t37;
    t72 = mEE.*t37;
    t73 = b2.^2;
    t74 = mEE.*t73;
    t75 = a1.*b1.*mDIST.*2.0;
    t76 = a1.*b1.*mEE.*2.0;
    t77 = a2.*b2.*mEE.*2.0;
    t78 = a2.*b0.*mDIST;
    t79 = a2.*b0.*mEE;
    t80 = b0.*b2.*mEE;
    t81 = t78+t79+t80;
    t82 = a1.*a3.*mEE;
    t83 = a3.*b1.*mEE;
    t84 = t82+t83;
    t85 = t56.*t84;
    t92 = a1.*b0.*mPROX;
    t93 = a1.*b0.*mDIST;
    t94 = a1.*b0.*mEE;
    t95 = b0.*b1.*mDIST;
    t96 = b0.*b1.*mEE;
    t97 = t92+t93+t94+t95+t96;
    t98 = t59.*t97;
    t112 = t61.*t81;
    t113 = a3.*b0.*mEE.*t63;
    t99 = IPROX+IDIST+IEE+t46+t51+t57+t64+t65+t66+t67+t68+t70+t71+t72+t74+t75+t76+t77+t98-t112-t113;
    t100 = a1.*a2.*mDIST;
    t101 = a1.*a2.*mEE;
    t102 = a2.*b1.*mDIST;
    t103 = a1.*b2.*mEE;
    t104 = a2.*b1.*mEE;
    t105 = b1.*b2.*mEE;
    t106 = t100+t101+t102+t103+t104+t105;
    t107 = t45.*t106;
    t108 = a2.*a3.*mEE;
    t109 = a3.*b2.*mEE;
    t110 = t108+t109;
    t111 = t50.*t110;
    t114 = IDIST+IEE+t51+t67+t68+t70+t74+t77+t85+t107;
    t115 = IEE+t70+t85+t111;
    t116 = IEE+t70+t111;
    InertiaS = reshape([t17,0.0,t30,-t86-t87-t88,-t88-t13.*t28,-t88,0.0,t17,t33,-t89-t90-t91,-t91-t24.*t28,-t91,t30,t33,IRED+IPROX+IDIST+IEE+t46+t51+t57+t64+t65+t66+t67+t68+t70+t71+t72+t74+t75+t76+t77+t59.*(a1.*b0.*mPROX.*2.0+a1.*b0.*mDIST.*2.0+a1.*b0.*mEE.*2.0+b0.*b1.*mDIST.*2.0+b0.*b1.*mEE.*2.0)+mPROX.*t36+mDIST.*t36+mEE.*t36-t61.*(a2.*b0.*mDIST.*2.0+a2.*b0.*mEE.*2.0+b0.*b2.*mEE.*2.0)-a3.*b0.*mEE.*t63.*2.0,t99,IDIST+IEE+t51+t67+t68+t70+t74+t77+t85+t107-t112-t113,IEE+t70+t85+t111-t113,-t7.*t8-t13.*t14-a3.*mEE.*t16,-t8.*t23-t14.*t24-a3.*mEE.*t25,t99,IPROX+IDIST+IEE+t46+t51+t57+t64+t65+t66+t67+t68+t70+t71+t72+t74+t75+t76+t77,t114,t115,-t13.*t28-a3.*mEE.*t16,-t24.*t28-a3.*mEE.*t25,IDIST+IEE+t51+t67+t68+t70+t74+t77+t85+t107-t61.*t81-a3.*b0.*mEE.*t63,t114,IDIST+IEE+t51+t67+t68+t70+t74+t77,t116,-a3.*mEE.*t16,-a3.*mEE.*t25,IEE+t70+t85+t111-a3.*b0.*mEE.*t63,t115,t116,IEE+t70],[6,6]);
end

== matlab function APF_Path_Planning_2023a/Thruster Control Code/Change RED Behavior/Calculate Thruster ON//OFF/MATLAB Function7 ==
  data: H output; thruster_dist2CG_RED parameter; F_red_X_nominal parameter; thrust_decay_factor input; F_red_Y_nominal parameter
function H   = MakeHWithDecay(thruster_dist2CG_RED,F_red_X_nominal, thrust_decay_factor, F_red_Y_nominal)


adjusted_thruster_dist2CG_RED = [thruster_dist2CG_RED(1);
                                 thruster_dist2CG_RED(2);
                                 thruster_dist2CG_RED(3);
                                 thruster_dist2CG_RED(4);
                                 thruster_dist2CG_RED(5);
                                 thruster_dist2CG_RED(6);
                                 thruster_dist2CG_RED(7);
                                 thruster_dist2CG_RED(8)];
                                 


Vec1 = [ -1
         -1
          0 
          0
          1
          1
          0
          0 ];
      
Vec2 = [  0
          0
          1
          1
          0
          0
         -1
         -1 ];
     
Vec3 = adjusted_thruster_dist2CG_RED./1000;

Mat1 = [Vec1, Vec2, Vec3]';

F_thrusters_RED = [F_red_X_nominal*thrust_decay_factor; F_red_X_nominal*thrust_decay_factor; F_red_Y_nominal*thrust_decay_factor; F_red_Y_nominal*thrust_decay_factor; F_red_X_nominal*thrust_decay_factor; F_red_X_nominal*thrust_decay_factor; F_red_Y_nominal*thrust_decay_factor; F_red_Y_nominal*thrust_decay_factor];

Mat2 = diag((F_thrusters_RED));

H    = Mat1*Mat2;

end

== matlab function APF_Path_Planning_2023a/Simulate Plant Dynamics/BLACK Dynamics/BLACK Dynamics Model/MATLAB Function ==
  data: control_inputs input; x_ddot output; mBLACK parameter; IBLACK parameter
function x_ddot = BLACK_dynamics(control_inputs, mBLACK, IBLACK)

%#codegen
% Fully define the size of x_ddot() for code generation:
x_ddot     = zeros(3,1);

% Extract the control inputs from the control_input vector:
Fx        = control_inputs(1);              % [N]
Fy        = control_inputs(2);              % [N]
Tz        = control_inputs(3);              % [N.m]

% Calculate the state acceleration vector:
x_ddot(1) = Fx/mBLACK;                      % [m/s^2]
x_ddot(2) = Fy/mBLACK;                      % [m/s^2]
x_ddot(3) = Tz/IBLACK;                      % [rad/s^2]

end

== matlab function APF_Path_Planning_2023a/Simulate Plant Dynamics/BLUE Dynamics/BLUE  Dynamics Model/MATLAB Function ==
  data: control_inputs input; x_ddot output; mBLUE parameter; IBLUE parameter
function x_ddot = BLUE_dynamics(control_inputs, mBLUE, IBLUE)%#codegen
% Fully define the size of x_ddot() for code generation:
x_ddot     = zeros(3,1);

% Extract the control inputs from the control_input vector:
Fx        = control_inputs(1);              % [N]
Fy        = control_inputs(2);              % [N]
Tz        = control_inputs(3);              % [N.m]

% Calculate the state acceleration vector:
x_ddot(1) = Fx/mBLUE;                      % [m/s^2]
x_ddot(2) = Fy/mBLUE;                      % [m/s^2]
x_ddot(3) = Tz/IBLUE;                      % [rad/s^2]

end

== matlab function APF_Path_Planning_2023a/Simulate Plant Dynamics/BLUE Dynamics/Sample and Hold Data to Match PhaseSpace (BLUE)/MATLAB Function ==
  data: TIME input; y output; SERVER input
function y = fcn(TIME, SERVER)

if mod(TIME,SERVER) == 0
    y = 1;
else
    y = 0;
end

== matlab function APF_Path_Planning_2023a/Simulate Plant Dynamics/RED and ARM Dynamics/RED Only/RED Dynamics/RED Dynamics Model/MATLAB Function ==
  data: control_inputs input; x_ddot output; mRED parameter; IRED parameter
    function x_ddot = RED_dynamics(control_inputs, mRED, IRED)
    
        %#codegen
        % Fully define the size of x_ddot() for code generation:
        x_ddot     = zeros(3,1);
        
        % Extract the servicer model parameters from the model_param vector defined
        % in initialize.m:
        
        % Extract the control inputs from the control_input vector:
        Fx        = control_inputs(1);              % [N]
        Fy        = control_inputs(2);              % [N]
        Tz        = control_inputs(3);              % [N.m]
        
        % Calculate the state acceleration vector:
        x_ddot(1) = Fx/mRED;                      % [m/s^2]
        x_ddot(2) = Fy/mRED;                      % [m/s^2]
        x_ddot(3) = Tz/IRED;                      % [rad/s^2]
    
    end

== matlab function APF_Path_Planning_2023a/Phase #2: Initial Position/Change RED Behavior/MATLAB Function2 ==
  data: error input; error_d input; u output; K_lqr parameter
function u = fcn(error,error_d,K_lqr)




u = K_lqr*([error(1);error(2);error(3);error_d(1);error_d(2);error_d(3)]);

end

== matlab function APF_Path_Planning_2023a/Phase #3: Experiment/Change RED Behavior/Sub-Phase #4/GDC/APF/GDC/MATLAB Function ==
  data: phi_tot output; phi_tot_grad output; state_red input; state_black input size=[6 1]; state_blue input; u output size=[3 1]; shape parameter; ka parameter; kr parameter; Q_a parameter; Q_b parameter; P_b parameter; r_hold parameter; Binv parameter; K_a parameter; psi parameter; sigma parameter; r_off parameter; Nmat parameter; state_desired output
function [phi_tot,phi_tot_grad,u,state_desired] = fcn(state_red,state_black,state_blue,shape,ka,kr,Q_a,Q_b,P_b,r_hold,Binv,K_a,psi,sigma,r_off,Nmat)

[phi_tot,phi_tot_grad,u,state_desired] = APF_func(state_red,state_black,state_blue,shape,ka,kr,Q_a,Q_b,P_b,r_hold,Binv,K_a,psi,sigma,r_off,Nmat);

== matlab function APF_Path_Planning_2023a/Thruster Control Code/Change BLACK Behavior/Calculate Thruster ON//OFF/MATLAB Function ==
  data: H output; thruster_dist2CG_BLACK parameter; F_thrusters_BLACK parameter
function H = MakeH(thruster_dist2CG_BLACK,F_thrusters_BLACK)

Vec1 = [ -1
         -1
          0 
          0
          1
          1
          0
          0 ];
      
Vec2 = [  0
          0
          1
          1
          0
          0
         -1
         -1 ];
     
Vec3 = thruster_dist2CG_BLACK./1000;

Mat1 = [Vec1, Vec2, Vec3]';

Mat2 = diag((F_thrusters_BLACK./2));

H    = Mat1*Mat2;

end

== matlab function APF_Path_Planning_2023a/Thruster Control Code/Change BLUE Behavior/Calculate Thruster ON//OFF/MATLAB Function1 ==
  data: H output; thruster_dist2CG_BLUE parameter; F_Blue_X_nominal parameter; thrust_decay_factor input; F_Blue_Y_nominal parameter
function H   = MakeHWithDecay(thruster_dist2CG_BLUE,F_Blue_X_nominal, thrust_decay_factor, F_Blue_Y_nominal)


adjusted_thruster_dist2CG_BLUE = [thruster_dist2CG_BLUE(1);
                                 thruster_dist2CG_BLUE(2);
                                 thruster_dist2CG_BLUE(3);
                                 thruster_dist2CG_BLUE(4);
                                 thruster_dist2CG_BLUE(5);
                                 thruster_dist2CG_BLUE(6);
                                 thruster_dist2CG_BLUE(7);
                                 thruster_dist2CG_BLUE(8)];
                                 


Vec1 = [ -1
         -1
          0 
          0
          1
          1
          0
          0 ];
      
Vec2 = [  0
          0
          1
          1
          0
          0
         -1
         -1 ];
     
Vec3 = adjusted_thruster_dist2CG_BLUE./1000;

Mat1 = [Vec1, Vec2, Vec3]';

F_thrusters_BLUE = [F_Blue_X_nominal*thrust_decay_factor; F_Blue_X_nominal*thrust_decay_factor; F_Blue_Y_nominal*thrust_decay_factor; F_Blue_Y_nominal*thrust_decay_factor; F_Blue_X_nominal*thrust_decay_factor; F_Blue_X_nominal*thrust_decay_factor; F_Blue_Y_nominal*thrust_decay_factor; F_Blue_Y_nominal*thrust_decay_factor];

Mat2 = diag((F_thrusters_BLUE));

H    = Mat1*Mat2;

end

== matlab function APF_Path_Planning_2023a/Thruster Control Code/Change BLUE Behavior/Calculate Thruster ON//OFF/MATLAB Function2 ==
  data: ThrustPer_Final output; ThrustPer input; PWMFreq parameter
function ThrustPer_Final  = ThrusterSat(ThrustPer, PWMFreq)

    ValveTime       = 0.007;
    TControl        = 1/PWMFreq;

    ThrustPer_Final = zeros(8,1);
    
    if max(ThrustPer) > 1
        ThrustPer_Sat = ThrustPer/max(ThrustPer);
    else
        ThrustPer_Sat = ThrustPer;
    end
    
    for i = 1:8
        if ThrustPer_Sat(i) > ValveTime/TControl 
            ThrustPer_Final(i) = ThrustPer_Sat(i);
        else
            ThrustPer_Final(i) = 0;
        end
    end


end

== matlab function APF_Path_Planning_2023a/Thruster Control Code/Change BLACK Behavior/Calculate Thruster ON//OFF/Rotate Forces to Inertial/Create Rotation Matrix ==
  data: Rz input; C_Ib output
function C_Ib = RotateFrame(Rz)

C_bI = [  cos(Rz) sin(Rz)
         -sin(Rz) cos(Rz) ];

C_Ib = inv(C_bI);

end

== matlab function APF_Path_Planning_2023a/Thruster Control Code/Change BLACK Behavior/Rotate Forces to Body/Create Rotation Matrix ==
  data: Rz input; C_bI output
function C_bI = RotateFrame(Rz)

C_bI = [  cos(Rz) sin(Rz)
         -sin(Rz) cos(Rz) ];

end

== matlab function APF_Path_Planning_2023a/Thruster Control Code/Change BLUE Behavior/Calculate Thruster ON//OFF/MATLAB Function ==
  data: H output; thruster_dist2CG_BLUE parameter; F_thrusters_BLUE parameter
function H = MakeH(thruster_dist2CG_BLUE,F_thrusters_BLUE)

Vec1 = [ -1
         -1
          0 
          0
          1
          1
          0
          0 ];
      
Vec2 = [  0
          0
          1
          1
          0
          0
         -1
         -1 ];
     
Vec3 = thruster_dist2CG_BLUE./1000;

Mat1 = [Vec1, Vec2, Vec3]';

Mat2 = diag((F_thrusters_BLUE./2));

H    = Mat1*Mat2;

end

== matlab function APF_Path_Planning_2023a/Thruster Control Code/Change BLACK Behavior/Calculate Thruster ON//OFF/MATLAB Function1 ==
  data: ThrustPer_Final output; ThrustPer input; PWMFreq parameter
function ThrustPer_Final  = ThrusterSat(ThrustPer, PWMFreq)

    ValveTime       = 0.007;
    TControl        = 1/PWMFreq;

    ThrustPer_Final = zeros(8,1);
    
    if max(ThrustPer) > 1
        ThrustPer_Sat = ThrustPer/max(ThrustPer);
    else
        ThrustPer_Sat = ThrustPer;
    end
    
    for i = 1:8
        if ThrustPer_Sat(i) > ValveTime/TControl 
            ThrustPer_Final(i) = ThrustPer_Sat(i);
        else
            ThrustPer_Final(i) = 0;
        end
    end


end

== matlab function APF_Path_Planning_2023a/Phase #3: Experiment/Change RED Behavior/Sub-Phase #4/GDC/APF/GDC/Subsystem1/Momentum/Momentum ==
  data: state_red input; phi_tot_grad input; v_prev input; path output size=3; v output size=3; momentum_eta parameter; momentum_gamma parameter
function [path, v] = momentum(state_red, phi_tot_grad, v_prev, momentum_eta, momentum_gamma)

% gamma = 0.9
v = -momentum_gamma.*v_prev-momentum_eta.*phi_tot_grad;
path = [state_red(1); state_red(2); state_red(3)] + v;

== matlab function APF_Path_Planning_2023a/Thruster Control Code/Change BLUE Behavior/Calculate Thruster ON//OFF/Rotate Forces to Inertial/Create Rotation Matrix ==
  data: Rz input; C_Ib output
function C_Ib = RotateFrame(Rz)

C_bI = [  cos(Rz) sin(Rz)
         -sin(Rz) cos(Rz) ];

C_Ib = inv(C_bI);

end

== matlab function APF_Path_Planning_2023a/Thruster Control Code/Change BLUE Behavior/Rotate Forces to Body/Create Rotation Matrix ==
  data: Rz input; C_bI output
function C_bI = RotateFrame(Rz)

C_bI = [  cos(Rz) sin(Rz)
         -sin(Rz) cos(Rz) ];

end

== matlab function APF_Path_Planning_2023a/Phase #2: Initial Position/Change BLACK Behavior/Hough Control/MATLAB Function2 ==
  data: Oy output; z input; Ox output
function [Oy, Ox]   = C3( z )
%C3 gives the rotation matrix about the z-axis for an angle 'z'
%   z - the angle about the z-axis which you rotate
%   A - the rotation matrix

Ox = [cos(z) sin(z); -sin(z) cos(z)]*[1;0];
Oy = [cos(z) sin(z); -sin(z) cos(z)]*[0;1];
end

== matlab function APF_Path_Planning_2023a/Phase #2: Initial Position/Change BLACK Behavior/Hough Control/MATLAB Function3 ==
  data: z input; Ox output
function Ox    = C3( z )
%C3 gives the rotation matrix about the z-axis for an angle 'z'
%   z - the angle about the z-axis which you rotate
%   A - the rotation matrix

Ox = [cos(z) sin(z); -sin(z) cos(z)]*[1;0];
end

== matlab function APF_Path_Planning_2023a/Phase #2: Initial Position/Change BLACK Behavior/Hough Control/MATLAB Function4 ==
  data: Oy input; e_out output; e_in input
function e_out = fcn(Oy, e_in)

a = sign(Oy'*e_in);
e_out = -a*norm(e_in);

== matlab function APF_Path_Planning_2023a/Phase #2: Initial Position/Change BLUE Behavior/Hough Control/MATLAB Function2 ==
  data: Oy output; z input; Ox output
function [Oy, Ox]   = C3( z )
%C3 gives the rotation matrix about the z-axis for an angle 'z'
%   z - the angle about the z-axis which you rotate
%   A - the rotation matrix

Ox = [cos(z) sin(z); -sin(z) cos(z)]*[1;0];
Oy = [cos(z) sin(z); -sin(z) cos(z)]*[0;1];
end

== matlab function APF_Path_Planning_2023a/Thruster Control Code/Change RED Behavior/Rotate Forces to Body/Create Rotation Matrix ==
  data: Rz input; C_bI output
function C_bI = RotateFrame(Rz)

C_bI = [  cos(Rz) sin(Rz)
         -sin(Rz) cos(Rz) ];

end

== matlab function APF_Path_Planning_2023a/Phase #2: Initial Position/Change BLUE Behavior/Hough Control/MATLAB Function3 ==
  data: z input; Ox output
function Ox    = C3( z )
%C3 gives the rotation matrix about the z-axis for an angle 'z'
%   z - the angle about the z-axis which you rotate
%   A - the rotation matrix

Ox = [cos(z) sin(z); -sin(z) cos(z)]*[1;0];
end

== matlab function APF_Path_Planning_2023a/Phase #2: Initial Position/Change BLUE Behavior/Hough Control/MATLAB Function4 ==
  data: Oy input; e_out output; e_in input
function e_out = fcn(Oy, e_in)

a = sign(Oy'*e_in);
e_out = -a*norm(e_in);

== matlab function APF_Path_Planning_2023a/Phase #2: Initial Position/Change RED Behavior/Hough Control/MATLAB Function2 ==
  data: Oy output; z input; Ox output
function [Oy, Ox]   = C3( z )
%C3 gives the rotation matrix about the z-axis for an angle 'z'
%   z - the angle about the z-axis which you rotate
%   A - the rotation matrix

Ox = [cos(z) sin(z); -sin(z) cos(z)]*[1;0];
Oy = [cos(z) sin(z); -sin(z) cos(z)]*[0;1];
end

== matlab function APF_Path_Planning_2023a/Phase #2: Initial Position/Change RED Behavior/Hough Control/MATLAB Function3 ==
  data: z input; Ox output
function Ox    = C3( z )
%C3 gives the rotation matrix about the z-axis for an angle 'z'
%   z - the angle about the z-axis which you rotate
%   A - the rotation matrix

Ox = [cos(z) sin(z); -sin(z) cos(z)]*[1;0];
end
